simulink model "DC_motor"  (R2025b)
settings: Solver=FixedStepAuto  StartTime=0.0  StopTime=sim_time  FixedStep=dt  MaxStep=dt  RelTol=1e-3
undefined symbols (not defined in the file): b, J, Kb, Kd, Ki, Kp, Kt, L, R, Torque, Vmax
libraries: slpidlib x1
settings Model: Creator=gianmarco  LastModifiedBy=gianmarco
settings DataIOCC: SaveFormat=Array

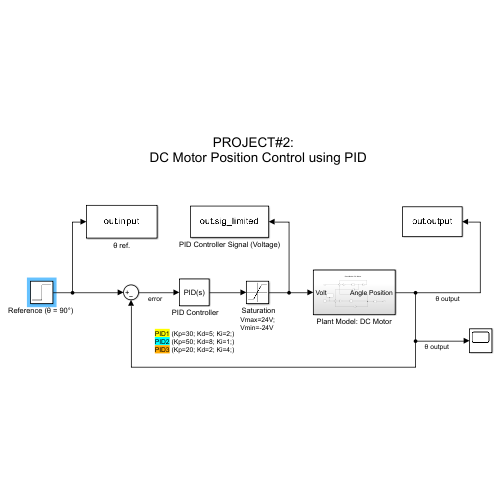
[thumbnail: Simulink's stored preview of the top-level diagram]
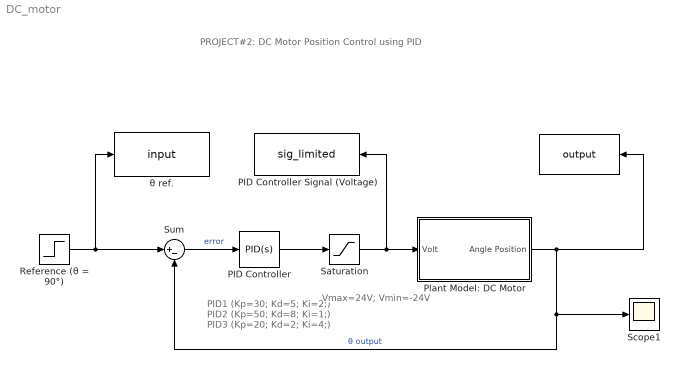
== system DC_motor ==
  note: PID1 (Kp=30; Kd=5; Ki=2;)
      | PID2 (Kp=50; Kd=8; Ki=1;)
      | PID3 (Kp=20; Kd=2; Ki=4;)
  note: PROJECT#2:
      | DC Motor Position Control using PID
  note: Vmax=24V;
      | Vmin=-24V
  " " : ToWorkspace  VariableName=output  SampleTime=-1
  " PID Controller" : slpidlib/PID Controller  Controller=PID  Form=Parallel  TimeDomain=Continuous-time  UseExternalTs=off  SampleTime=-1  IntegratorMethod=Forward Euler  FilterMethod=Forward Euler  ControllerParametersSource=internal  P=10  I=Kp  UseKiTs=off  D=Kd  UseExternalDerivativeSource=off  N=Ki  UseFilter=on  TunerSelectOption=Transfer Function Based (PID Tuner App)  InitialConditionSource=internal  InitialConditionForIntegrator=0  InitialConditionForFilter=0  DifferentiatorICPrevScaledInput=0  ExternalReset=none  TrackingMode=off  Kt=1  LimitOutput=off  SatLimitsSource=internal  UpperSaturationLimit=inf  LowerSaturationLimit=-inf  LinearizeAsGain=on  AntiWindupMode=none  Kb=1  LimitIntegrator=off  UpperIntegratorSaturationLimit=inf  LowerIntegratorSaturationLimit=-inf  POutMin=[]  POutMax=[]  IOutMin=[]  IOutMax=[]  DOutMin=[]  DOutMax=[]  NOutMin=[]  NOutMax=[]  SumOutMin=[]  SumOutMax=[]  SaturationOutMin=[]  SaturationOutMax=[]  PParamMin=[]  PParamMax=[]  IParamMin=[]  IParamMax=[]  DParamMin=[]  DParamMax=[]  NParamMin=[]  NParamMax=[]  KbParamMin=[]  KbParamMax=[]  KtParamMin=[]  KtParamMax=[]  KbOutMin=[]  KbOutMax=[]  KtOutMin=[]  KtOutMax=[]  IntegratorOutMin=[]  IntegratorOutMax=[]  FilterOutMin=[]  FilterOutMax=[]  SumI1OutMin=[]  SumI1OutMax=[]  SumI2OutMin=[]  SumI2OutMax=[]  SumI3OutMin=[]  SumI3OutMax=[]  SumI4OutMin=[]  SumI4OutMax=[]  SumDOutMin=[]  SumDOutMax=[]  DifferentiatorOutMin=[]  DifferentiatorOutMax=[]  FilterDiffOutCoefMin=[]  FilterDiffOutCoefMax=[]  ReciprocalOutMin=[]  ReciprocalOutMax=[]  SumDenOutMin=[]  SumDenOutMax=[]  SumNumOutMin=[]  SumNumOutMax=[]  DivideOutMin=[]  DivideOutMax=[]  UdiffTsProdOutMin=[]  UdiffTsProdOutMax=[]  NTsProdOutMin=[]  NTsProdOutMax=[]  UintegralTsProdOutMin=[]  UintegralTsProdOutMax=[]  UngainTsProdOutMin=[]  UngainTsProdOutMax=[]  ClampingZeroOutDataTypeStr=Inherit: Inherit via back propagation  ClampingZeroOutMin=[]  ClampingZeroOutMax=[]  FilterDenConstantOutDataTypeStr=Inherit: Inherit via back propagation  FilterDenConstantOutMin=[]  FilterDenConstantOutMax=[]  PCopyOutDataTypeStr=Inherit: Inherit via back propagation  PCopyOutMin=[]  PCopyOutMax=[]  NCopyOutDataTypeStr=Inherit: Inherit via back propagation  NCopyOutMin=[]  NCopyOutMax=[]  IntegratorContinuousStateAttributes=''  IntegratorStateMustResolveToSignalObject=off  IntegratorRTWStateStorageClass=Auto  FilterContinuousStateAttributes=''  FilterStateMustResolveToSignalObject=off  FilterRTWStateStorageClass=Auto  ParallelPVariant=InternalParameters  IdealPVariant=Disabled  IVariant=InternalParameters  DVariant=InternalParameters  IntegratorVariant=Continuous  SatVariant=Disabled  AWVariant=Passthrough  PCopyVariant=Disabled  TRVariant=Disabled  FdbkBlocksVariant=Forward  IdealPFdbkVariant=Disabled  SatFdbkVariant=Disabled  DerivativeFilterVariant=ContFilter  NVariant=InternalParameters  NCopyVariant=Disabled  FilterICVariant=InternalICsFilter  IntegratorICVariant=InternalICs  ExternalResetVariant=Disabled  TRSumVariant=Passthrough  SumFdbkVariant=Disabled  SumVariant=Sum_PID  TsampFilterVariant=InternalTs  TsampNgainVariant=Passthrough  TsampIntegralVariant=Disabled_SignalSpec  ExternalSaturationOutDataTypeStr=Inherit: Same as second input  DerivativeSourceVariant=ErrorSignal  PreIntVariant=InternalPreInt
  " Saturation" : Saturate  UpperLimit=Vmax  LowerLimit=-Vmax
  PID Controller Signal (Voltage) : ToWorkspace  VariableName=sig_limited  SampleTime=-1
  Plant Model: DC Motor : Subsystem
  "Reference (θ = 90°) " : Step  After=pi/2  SampleTime=0
  Scope1 : Scope
      settings: ActiveDisplayYMinimum=-1  ActiveDisplayYMaximum=1
  Sum : Sum  Inputs=|+-
  θ ref. : ToWorkspace  VariableName=input  SampleTime=-1
  wires:
  "Reference (θ = 90°) "/1 -> Sum/1, θ ref./1
  Plant Model: DC Motor/1(Angle Position) -> " "/1, Scope1/1, Sum/2  "θ output"
  " PID Controller"/1 -> " Saturation"/1
  Sum/1 -> " PID Controller"/1  "error"
  " Saturation"/1 -> Plant Model: DC Motor/1(Volt), PID Controller Signal (Voltage)/1

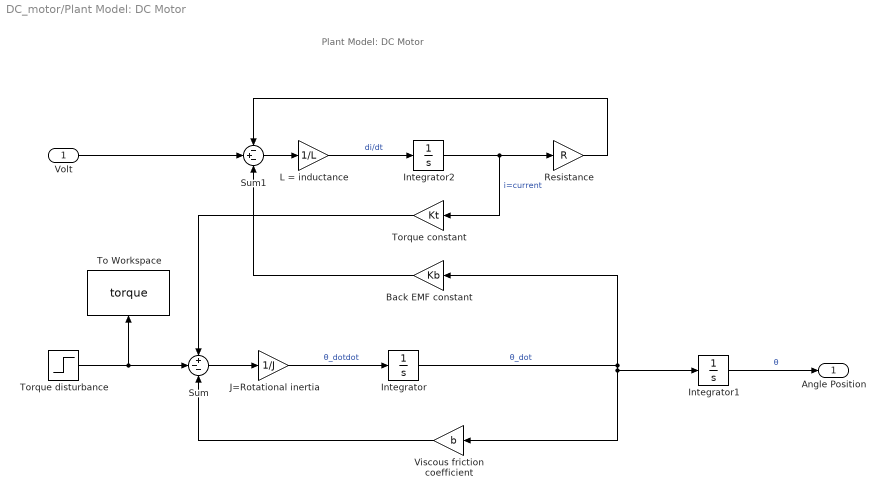
== system DC_motor/Plant Model: DC Motor ==
  note: Plant Model: DC Motor
  Volt : Inport
  "  Integrator" : Integrator
  " Integrator1" : Integrator
  " Resistance" : Gain  Gain=R
  Back EMF constant : Gain  Gain=Kb
  Integrator2 : Integrator
  J=Rotational inertia : Gain  Gain=1/J
  L = inductance : Gain  Gain=1/L
  Sum : Sum  Inputs=+--
  Sum1 : Sum  Inputs=-+-
  To Workspace : ToWorkspace  VariableName=torque  SampleTime=-1
      settings: Save2DSignal=2-D array (concatenate along first dimension)
  Torque constant : Gain  Gain=Kt
  Torque disturbance : Step  After=Torque  SampleTime=0
  Viscous friction coefficient : Gain  Gain=b
  Angle Position : Outport
  wires:
  L = inductance/1 -> Integrator2/1  "di/dt"
  " Integrator1"/1 -> Angle Position/1  "θ"
  Sum/1 -> J=Rotational inertia/1
  "  Integrator"/1 -> Viscous friction coefficient/1, " Integrator1"/1, Back EMF constant/1  "θ_dot"
  Volt/1 -> Sum1/2
  Integrator2/1 -> Torque constant/1, " Resistance"/1  "i=current"
  " Resistance"/1 -> Sum1/1
  Viscous friction coefficient/1 -> Sum/3
  J=Rotational inertia/1 -> "  Integrator"/1  "θ_dotdot"
  Back EMF constant/1 -> Sum1/3
  Sum1/1 -> L = inductance/1
  Torque constant/1 -> Sum/1
  Torque disturbance/1 -> To Workspace/1, Sum/2
